simulink model "untitled"  (R2018a)
settings: Solver=VariableStepAuto  StartTime=0.0  StopTime=inf  RelTol=1e-3
undefined symbols (not defined in the file): gray, Rec, SDTV
libraries: visionanalysis x2, visionconversions x1, visiongeotforms x1, dspvision x1
settings Model: Creator=놀러와마이홈  LastModifiedBy=놀러와마이홈

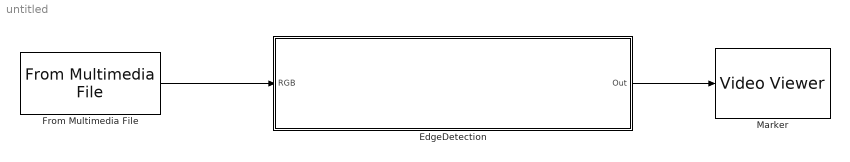
== system untitled ==
  EdgeDetection : Subsystem
  From Multimedia File : dspvision/From Multimedia File  inputFilename=C:\Users\놀러와마이홈\Downloads\Video\Video1.mp4  loop=on  numPlays=inf  outputStreams=Video only  videoDataType=single  audioDataType=int16  inheritSampleTime=on  userDefinedSampleTime=1/30  noAudioOutput=off  isIntensityVideo=off  fourcc=RGB  colorVideoFormat=One multidimensional signal  outputEOF=off  dataOrg=Column-major  audioFrameSize=1024  computeAudioFrameSize=off  outSamplingMode=Sample based
      settings: SourceProductBaseCode=VP
  Marker : VideoViewer  colormapValue=gray(256)  FigPos=[1.66666666666667 677.333333333333 638.666666666667 574.666666666667]
  wires:
  From Multimedia File/1 -> EdgeDetection/1(RGB)
  EdgeDetection/1(Out) -> Marker/1

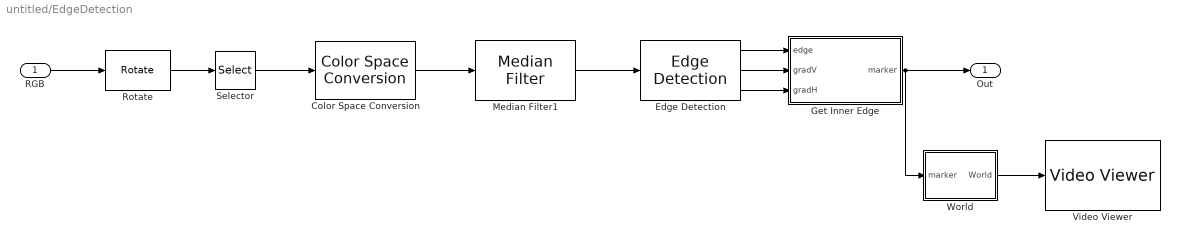
== system untitled/EdgeDetection ==
  RGB : Inport
  Color Space Conversion : visionconversions/Color Space  Conversion  conversion=Obsolete  conversionActive=R'G'B' to intensity  wp_str=D65  rec=Rec. 601 (SDTV)  sys=1125/60/2:1  imagePorts=One multidimensional signal
      settings: SourceProductName=Computer Vision System Toolbox
  Edge Detection : visionanalysis/Edge Detection  method=Sobel  outputType=Binary image and gradient components  userDefinedThreshold=off  thresholdSource=Specify via dialog  threshold=4  thresholdTuning=35  edgeThinning=on  threshold_canny=[0.25 0.60]  autoPercent=70  sigma=1  roundingMode=Floor  overflowMode=off  prodOutputMode=Binary point scaling  prodOutputWordLength=32  prodOutputFracLength=8  prodOutputSlope=2^-8  accumSlope=2^-8  outputSlope=2^-4
      settings: SourceProductName=Computer Vision System Toolbox  SourceProductBaseCode=VP
  Get Inner Edge : MATLAB Function  TreatAsAtomicUnit=on
  Median Filter1 : visionanalysis/Median Filter  nghbood=[3 3]  outSize=Same as input port I  padType=Constant  padSrc=Specify via dialog  padVal=0  roundingMode=Floor  overflowMode=off
      settings: SourceProductName=Computer Vision System Toolbox  SourceProductBaseCode=VP
  Rotate : visiongeotforms/Rotate  outSizeR=Expanded to fit rotated input image  src_angle=Specify via dialog  unit_angle=Degrees  angle=pi  maxAngle=pi  dispImage=Top-left corner  method=Table lookup  fillVal=0  interpMethod=Bilinear  prodOutputMode=Binary point scaling  prodOutputWordLength=32  prodOutputFracLength=10  roundingMode=Nearest  overflowMode=on
      settings: SourceProductName=Computer Vision System Toolbox
  Selector : Selector  NumberOfDimensions=3  InputPortWidth=3  IndexOptions=Index vector (dialog),Select all,Select all  Indices=581:1080,1,1  OutputSizes=1,1,1
  Video Viewer : VideoViewer  colormapValue=gray(256)  FigPos=[641.666666666667 677.333333333333 638.666666666667 574.666666666667]
  World : MATLAB Function  TreatAsAtomicUnit=on
  Out : Outport
  wires:
  RGB/1 -> Rotate/1
  Rotate/1 -> Selector/1
  Selector/1 -> Color Space Conversion/1
  Color Space Conversion/1 -> Median Filter1/1
  Median Filter1/1 -> Edge Detection/1
  Edge Detection/1 -> Get Inner Edge/1(edge)
  Edge Detection/2 -> Get Inner Edge/2(gradV)
  Edge Detection/3 -> Get Inner Edge/3(gradH)
  Get Inner Edge/1(marker) -> World/1(marker), Out/1
  World/1(World) -> Video Viewer/1

== matlab function untitled/EdgeDetection/World ==
  data: marker input; World output
function World = fcn(marker)
%% Homography Matrix
% Pw=inv(h) * Pu

  h=[-46.84381893306346, 70.98490813576517, -246.2952904288011;
 -17.38476832232272, 9.621414012831043, -8435.459745198856;
 -0.03962156294964917, 0.007832870639782169, 1];

% World coordinates
World=zeros(500,1920,'logical');
% A is getting marker pixel coordinates
% B is Pw
% Homography 연산을 통해 얻어낸 좌표를 (a; b; c)라고 할 때
% World 좌표는 (a/c b/c)으로 나타나므로 C라는 행렬을 선언하여 
% 위의 a/c. b/c 계산 된 값을 저장하고 World 픽셀에 대입
A=ones(3,1);
C=zeros(1,2);
%% 
for i=1:500
    for j=1:1920
        % marker에 해당 되는 픽셀의 값이 0일때
        if marker(i,j)==false
            continue;
        end
        % marker에 해당 되는 픽셀의 값이 1일때
        if marker(i,j)==true
        A(1,1)=i;
        A(2,1)=j;
        % Homography 연산
        B=inv(h)*A;
        C(1,1)=fix(B(1,1)/B(3,1));
        C(1,2)=fix(B(2,1)/B(3,1));
        % 디버깅했을 때 예측 불가능 한 수들은 World 좌표에서
        % (290,290)처리 (왜 나오는지는 확인 하지 못했습니다.)
        if C(1,1)>300 || C(1,2) >300 || C(1,1) < 0 || C(1,2) < 0
            C(1,1)=290;
            C(1,2)=290;
        end
        % Pixel에서는 음수가 나올 수 없으므로 일단은 절대값처리하여
        % 값이 제대로 출력되는 지 확인
        if C(1,1) < 0 || C(1,2) < 0
            C(1,1)=abs(C(1,1));
            C(1,2)=abs(C(1,2));
        end
        World(C(1),C(2))=true;
        end
    end
   
end

end

== matlab function untitled/EdgeDetection/Get Inner Edge ==
  data: edge input; marker output; gradV input; gradH input
%% Find Rising or Falling edge
%Initializing Pixel (Pixel to zero)
function marker = fcn(edge, gradV, gradH)

marker = zeros(size(edge),'logical');
A=zeros(1,2);
% ROI Rows
for i=1:500
% ROI Column
    for j=1:1920
%% if Pixel is Black, marker is 0(False)
        if edge(i,j)==false
        continue;
        end
 %% Find Inner Edge 
        ang=atan2(gradV(i,j),gradH(i,j));
    %    if abs(ang)<pi/9 || abs(ang)>16/18*pi
    %        continue;
    %    end
    %    if abs(ang)>pi/2 && abs(ang)<pi
    %        continue;        
    %    end    
   
 %% else(Inner Edge), marker is 1(True)
        marker(i,j)=true;
    end
end
